simulink model "task2"  (R2022b)
settings: Solver=FixedStepAuto  StartTime=0.0  StopTime=7  RelTol=1e-8
undefined symbols (not defined in the file): a0, a1, a2, k0, k1, T, y0, y1
settings Model: Creator=anton  LastModifiedBy=anton
settings DataIOCC: ExternalInput=data

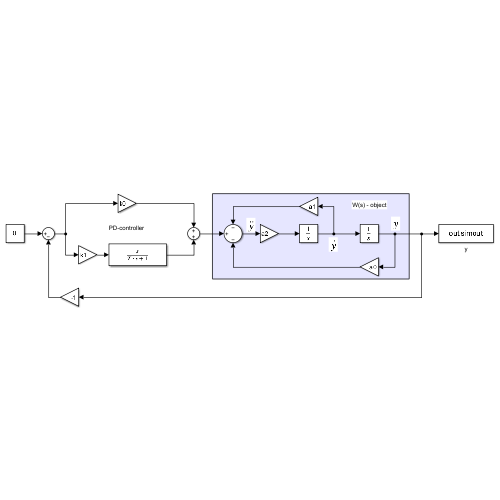
[thumbnail: Simulink's stored preview of the top-level diagram]
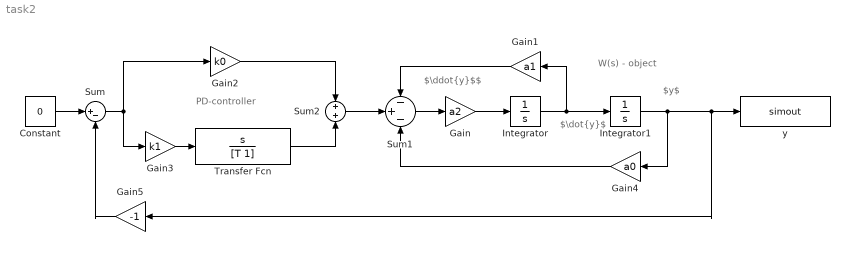
== system task2 ==
  note: PD-controller
  note: W(s) - object
  note: $\ddot{y}$$
  note: $\dot{y}$
  note: $y$
  Constant : Constant  Value=0
  Gain : Gain  Gain=a2
  Gain1 : Gain  Gain=a1
  Gain2 : Gain  Gain=k0
  Gain3 : Gain  Gain=k1
  Gain4 : Gain  Gain=a0
  Gain5 : Gain  Gain=-1
  Integrator : Integrator  InitialCondition=y1
  Integrator1 : Integrator  InitialCondition=y0
  Sum : Sum  Inputs=|+-
  Sum1 : Sum  Inputs=-+-
  Sum2 : Sum
  Transfer Fcn : TransferFcn  Numerator=[1 0]  Denominator=[T 1]
  y : ToWorkspace  VariableName=simout  SaveFormat=Timeseries  SampleTime=-1
  wires:
  Constant/1 -> Sum/1
  Gain3/1 -> Transfer Fcn/1
  Gain2/1 -> Sum2/1
  Sum/1 -> Gain2/1, Gain3/1
  Integrator1/1 -> Gain5/1, y/1, Gain4/1
  Gain/1 -> Integrator/1
  Integrator/1 -> Gain1/1, Integrator1/1
  Sum1/1 -> Gain/1
  Gain4/1 -> Sum1/3
  Sum2/1 -> Sum1/2
  Gain1/1 -> Sum1/1
  Transfer Fcn/1 -> Sum2/2
  Gain5/1 -> Sum/2
